simulink model "Test - Copy"  (R2019b)
settings: Solver=FixedStepAuto  StartTime=0.0  StopTime=10.0  FixedStep=0.005  RelTol=1e-3
undefined symbols (not defined in the file or in its folder): obj
settings Model: Creator=mecha  LastModifiedBy=mecha

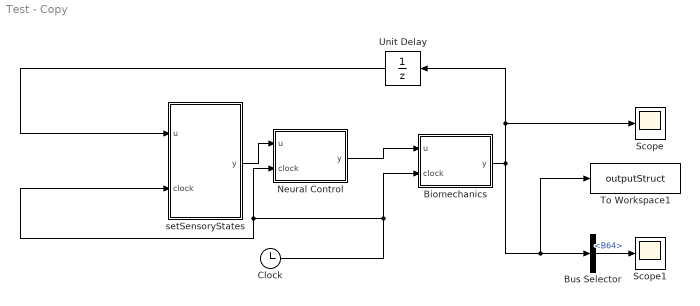
== system Test - Copy ==
  Biomechanics : MATLAB Function  TreatAsAtomicUnit=on
  Bus Selector : BusSelector  OutputSignals=B64
  Clock : Clock
  Neural Control : MATLAB Function  TreatAsAtomicUnit=on
  Scope : Scope
  Scope1 : Scope
  To Workspace1 : ToWorkspace  VariableName=outputStruct  SaveFormat=Timeseries  SampleTime=-1
  Unit Delay : UnitDelay  InitialCondition=obj  SampleTime=-1  HasFrameUpgradeWarning=on
  setSensoryStates : MATLAB Function  TreatAsAtomicUnit=on
  wires:
  Clock/1 -> Neural Control/2(clock), setSensoryStates/2(clock), Biomechanics/2(clock)
  Neural Control/1(y) -> Biomechanics/1(u)
  Biomechanics/1(y) -> Scope/1, Unit Delay/1, To Workspace1/1, Bus Selector/1
  setSensoryStates/1(y) -> Neural Control/1(u)
  Unit Delay/1 -> setSensoryStates/1(u)
  Bus Selector/1 -> Scope1/1  "<B64>"

== matlab function Test - Copy/Biomechanics ==
  data: u input Bus: AplysiaBus; y output Bus: AplysiaBus; clock input
function y = fcn(u, clock)
y=u;
%% Initialize internal tracking variables
tc=clock;
x_gh = u.x_g-u.x_h;
%initialize to avoid validation error upon build
F_f_g = 0;
F_f_h=0;
A11=0;
A12=0;
A21=0;
A22=0;
B1=0;
B2=0;
%% Biomechanics

%% Grasper Forces
%all forces in form F = Ax+b
F_I2 = u.max_I2*u.T_I2*[1,-1]*[u.x_h;u.x_g] + u.max_I2*u.T_I2*1; %FI2 = FI2_max*T_I2*(1-(xg-xh))
F_I3 = u.max_I3*u.T_I3*[-1,1]*[u.x_h;u.x_g]-u.max_I3*u.T_I3*0; %FI3 = FI3_max*T_I3*((xg-xh)-0)
F_hinge = (x_gh>0.5)*u.max_hinge*u.T_hinge*[-1,1]*[u.x_h;u.x_g]-(x_gh>0.5)*u.max_hinge*u.T_hinge*0.5; %F_hinge = [hinge stretched]*F_hinge_Max*T_hinge*((xg-xh)-0.5)
F_sp_g = u.K_sp_g*[1,-1]*[u.x_h;u.x_g]+u.K_sp_g*u.x_gh_ref; %F_sp,g = K_g((xghref-(xg-xh))

F_I4 = u.max_I4*u.P_I4;
F_I3_ant = u.max_I3ant*u.P_I3_anterior*[1,-1]*[u.x_h;u.x_g]+u.max_I3ant*u.P_I3_anterior*1;%: pinch force

%calculate F_f for grasper
if(u.fixation_type == 0) %object is not fixed to a contrained surface
    %F_g = F_I2+F_sp_g-F_I3-F_hinge; %if the object is unconstrained it does not apply a resistive force back on the grasper. Therefore the force is just due to the muscles

    A2 = 1/u.c_g*(u.max_I2*u.T_I2*[1,-1]+u.K_sp_g*[1,-1]-u.max_I3*u.T_I3*[-1,1]-u.max_hinge*u.T_hinge*(x_gh>0.5)*[-1,1]);
    B2 = 1/u.c_g*(u.max_I2*u.T_I2*1+u.K_sp_g*u.x_gh_ref+u.max_I3*u.T_I3*0+(x_gh>0.5)*u.max_hinge*u.T_hinge*0.5);

    A21 = A2(1);
    A22 = A2(2);

    %the force on the object is approximated based on the friction
    if(abs(F_I2+F_sp_g-F_I3-F_hinge) <= abs(u.mu_s_g*F_I4)) % static friction is true
        %disp('static')
        F_f_g = -u.sens_mechanical_grasper*(F_I2+F_sp_g-F_I3-F_hinge);
        y.grasper_friction_state = 1;
    else
        %disp('kinetic')
        F_f_g = u.sens_mechanical_grasper*u.mu_k_g*F_I4;
        %specify sign of friction force
        F_f_g = -(F_I2+F_sp_g-F_I3-F_hinge)/abs(F_I2+F_sp_g-F_I3-F_hinge)*F_f_g;
        y.grasper_friction_state = 0;
    end

elseif (u.fixation_type == 1) %object is fixed to a contrained surface
    if u.unbroken
        if(abs(F_I2+F_sp_g-F_I3-F_hinge) <= abs(u.mu_s_g*F_I4)) % static friction is true
            %disp('static')
            F_f_g = -u.sens_mechanical_grasper*(F_I2+F_sp_g-F_I3-F_hinge);
            %F_g = F_I2+F_sp_g-F_I3-F_hinge + F_f_g;
            y.grasper_friction_state = 1;

            %identify matrix components for semi-implicit integration
            A21 = 0;
            A22 = 0;
            B2 = 0;

        else
            %disp('kinetic')
            F_f_g = -sign(F_I2+F_sp_g-F_I3-F_hinge)*u.sens_mechanical_grasper*u.mu_k_g*F_I4;
            %specify sign of friction force
            %F_g = F_I2+F_sp_g-F_I3-F_hinge + F_f_g;
            y.grasper_friction_state = 0;


            %identify matrix components for semi-implicit integration
            A2 = 1/u.c_g*(u.max_I2*u.T_I2*[1,-1]+u.K_sp_g*[1,-1]-u.max_I3*u.T_I3*[-1,1]-u.max_hinge*u.T_hinge*(x_gh>0.5)*[-1,1]);
            B2 = 1/u.c_g*(u.max_I2*u.T_I2*1+u.K_sp_g*u.x_gh_ref+u.max_I3*u.T_I3*0+(x_gh>0.5)*u.max_hinge*u.T_hinge*0.5+F_f_g);

            A21 = A2(1);
            A22 = A2(2);

        end
    else
        %F_g = F_I2+F_sp_g-F_I3-F_hinge; %if the object is unconstrained it does not apply a resistive force back on the grasper. Therefore the force is just due to the muscles

        A2 = 1/u.c_g*(u.max_I2*u.T_I2*[1,-1]+u.K_sp_g*[1,-1]-u.max_I3*u.T_I3*[-1,1]-u.max_hinge*u.T_hinge*(x_gh>0.5)*[-1,1]);
        B2 = 1/u.c_g*(u.max_I2*u.T_I2*1+u.K_sp_g*u.x_gh_ref+u.max_I3*u.T_I3*0+(x_gh>0.5)*u.max_hinge*u.T_hinge*0.5);

        A21 = A2(1);
        A22 = A2(2);

        %the force on the object is approximated based on the friction
        if(abs(F_I2+F_sp_g-F_I3-F_hinge) <= abs(u.mu_s_g*F_I4)) % static friction is true
            %disp('static')
            F_f_g = -u.sens_mechanical_grasper*(F_I2+F_sp_g-F_I3-F_hinge);
            y.grasper_friction_state = 1;
        else
            %disp('kinetic')
            F_f_g = u.sens_mechanical_grasper*u.mu_k_g*F_I4;
            %specify sign of friction force
            F_f_g = -(F_I2+F_sp_g-F_I3-F_hinge)/abs(F_I2+F_sp_g-F_I3-F_hinge)*F_f_g;
            y.grasper_friction_state = 0;
        end
    end
end
%[j*dt position_grasper_relative I2 F_sp I3 hinge GrapserPressure_last F_g]

%% Body Forces
%all forces in the form F = Ax+b
F_sp_h = u.K_sp_h*[-1,0]*[u.x_h;u.x_g]+u.x_h_ref*u.K_sp_h;
%all muscle forces are equal and opposite
if(u.fixation_type == 0)     %object is not constrained
    %F_h = F_sp_h; %If the object is unconstrained it does not apply a force back on the head. Therefore the force is just due to the head spring.

    A1 = 1/u.c_h*u.K_sp_h*[-1,0];
    B1 = 1/u.c_h*u.x_h_ref*u.K_sp_h;

    A11 = A1(1);
    A12 = A1(2);

    if(abs(F_sp_h+F_f_g) <= abs(u.mu_s_h*F_I3_ant)) % static friction is true
        %disp('static2')
        F_f_h = -u.sens_mechanical_grasper*(F_sp_h+F_f_g); %only calculate the force if an object is actually present
        y.jaw_friction_state = 1;
    else
        %disp('kinetic2')
        F_f_h = -sign(F_sp_h+F_f_g)*u.sens_mechanical_grasper*u.mu_k_h*F_I3_ant; %only calculate the force if an object is actually present
        y.jaw_friction_state = 0;
    end
elseif (u.fixation_type == 1)
    %calcuate friction due to jaws
    if u.unbroken %if the seaweed is intact
        if(abs(F_sp_h+F_f_g) <= abs(u.mu_s_h*F_I3_ant)) % static friction is true
            %disp('static2')
            F_f_h = -u.sens_mechanical_grasper*(F_sp_h+F_f_g); %only calculate the force if an object is actually present
            %F_h = F_sp_h+F_f_g + F_f_h;
            y.jaw_friction_state = 1;

            A11 = 0;
            A12 = 0;
            B1 = 0;

        else
            %disp('kinetic2')
            F_f_h = -sign(F_sp_h+F_f_g)*u.sens_mechanical_grasper*u.mu_k_h*F_I3_ant; %only calculate the force if an object is actually present
            %F_h = F_sp_h+F_f_g + F_f_h;

            y.jaw_friction_state = 0;

            if (y.grasper_friction_state == 1) %object is fixed and grasper is static  
            % F_f_g = -mechanical_in_grasper*(F_I2+F_sp_g-F_I3-F_Hi);
                A1 = 1/u.c_h*(u.K_sp_h*[-1,0]+(-u.sens_mechanical_grasper*(u.max_I2*u.T_I2*[1,-1]+u.K_sp_g*[1,-1]-u.max_I3*u.T_I3*[-1,1]-u.max_hinge*u.T_hinge*(x_gh>0.5)*[-1,1]))...
                    -sign(F_sp_h+F_f_g)*u.sens_mechanical_grasper*u.mu_k_h*u.max_I3ant*u.P_I3_anterior*[1,-1]);
                B1 = 1/u.c_h*(u.x_h_ref*u.K_sp_h+(-u.sens_mechanical_grasper*(u.max_I2*u.T_I2*1+u.K_sp_g*u.x_gh_ref+u.max_I3*u.T_I3*0+(x_gh>0.5)*u.max_hinge*u.T_hinge*0.5))...
                    -sign(F_sp_h+F_f_g)*u.sens_mechanical_grasper*u.mu_k_h*u.max_I3ant*u.P_I3_anterior*1);

            else %both are kinetic
            %F_f_g = -sign(F_I2+F_sp_g-F_I3-F_Hi)*mechanical_in_grasper*mu_k_g*F_I4;
                A1 = 1/u.c_h*(u.K_sp_h*[-1,0]-sign(F_sp_h+F_f_g)*u.sens_mechanical_grasper*u.mu_k_h*u.max_I3ant*u.P_I3_anterior*[1,-1]);
                B1 = 1/u.c_h*(u.x_h_ref*u.K_sp_h-sign(F_I2+F_sp_g-F_I3-F_hinge)*u.sens_mechanical_grasper*u.mu_k_g*F_I4...
                    -sign(F_sp_h+F_f_g)*u.sens_mechanical_grasper*u.mu_k_h*u.max_I3ant*u.P_I3_anterior*1);                
            end
            A11= A1(1);
            A12 = A1(2);
        end
    else % if the seaweed is broken the jaws act as if unconstrained
        if(abs(F_sp_h+F_f_g) <= abs(u.mu_s_h*F_I3_ant)) % static friction is true
        %disp('static2')
            F_f_h = -u.sens_mechanical_grasper*(F_sp_h+F_f_g); %only calculate the force if an object is actually present
            y.jaw_friction_state = 1;
        else
            %disp('kinetic2')
            F_f_h = -sign(F_sp_h+F_f_g)*u.sens_mechanical_grasper*u.mu_k_h*F_I3_ant; %only calculate the force if an object is actually present
            y.jaw_friction_state = 0;
        end

        A1 = 1/u.c_h*u.K_sp_h*[-1,0];
        B1 = 1/u.c_h*u.x_h_ref*u.K_sp_h;

        A11 = A1(1);
        A12 = A1(2);
        y.jaw_friction_state = 0;

    end
end
%[position_buccal_last F_h F_sp I3 hinge force_pinch F_H]


%% Integrate body motions
%uncomment to remove periphery
%F_g = 0;
%F_H = 0;

A = [A11,A12;A21,A22];
B = [B1;B2];

x_last = [u.x_h;u.x_g];

x_new = 1/(1-u.TimeStep*trace(A))*((eye(2)+u.TimeStep*[-A22,A12;A21,-A11])*x_last+u.TimeStep*B);

y.x_g = x_new(2); 
y.x_h = x_new(1);

%% calculate force on object
y.force_on_object = F_f_g+F_f_h;

%check if seaweed is broken
if (u.fixation_type ==1)
    if (y.force_on_object>u.seaweed_strength)
        u.unbroken = 0;
    end
    %check to see if a new cycle has started
    x_gh_next = y.x_g-y.x_h;

    if (~u.unbroken && x_gh <0.3 && x_gh_next>x_gh)%x_gh<0.3)
       y.unbroken = 1; 
    end
y.force_on_object= y.unbroken*y.force_on_object;
end










end

== matlab function Test - Copy/Neural Control ==
  data: u input Bus: AplysiaBus; y output Bus: AplysiaBus; clock input
function y = fcn(u, clock)
y=u
%% Initialize internal tracking variables
tc=clock;

%j=1;

% u.CBI3_stimON = 0;
% u.CBI3_stimOFF = 0;
% u.CBI3_refractory = 0;
% u.B40B30_offTime = 0;
% u.unbroken = 1; %tracking variable to keep track of seaweed being broken off during feeding



x_gh = u.x_g-u.x_h;

%% Update Metacerebral cell: 
% assume here feeding arousal continues
% indefinitely, once started. 
%{
MCC is active IF
    General Food arousal is on
%}

y.MCC=u.MCC;

%% Update CBI-2
%{
CBI2 is active IF
    MCC is on 
    AND (
        (Mechanical Stimulation at Lips AND Chemical Stimulation at Lips AND No mechanical stimuli in grasper)
        OR 
        (Mechanical in grasper and no Chemical Stimulation at Lips)
        OR
        (B4/B5 is firing strongly (>=2)))
%}

%CBI2 - updated 6/7/2020
%with hypothesized connections from B4/B5
if (u.use_hypothesized_connections ==1)
     y.CBI2 = (u.stim_CBI2==0)*... if electrode above CBI-2 is off, do this:
         u.MCC*(~u.B64)*((u.sens_mechanical_lips && u.sens_chemical_lips &&(~u.sens_mechanical_grasper))||(u.sens_mechanical_grasper &&(~u.sens_chemical_lips))||(u.B4B5>=2))+...
         (u.stim_CBI2==1);
else
%without hypothesized connections from B4/B5
    y.CBI2 = (u.stim_CBI2==0)*... if electrode above CBI-2 is off, do this:
        u.MCC*(~u.B64)*((u.sens_mechanical_lips && u.sens_chemical_lips &&(~u.sens_mechanical_grasper))||(u.sens_mechanical_grasper&&(~u.sens_chemical_lips)))+...
        (u.stim_CBI2==1);
end

%% Update CBI-3
% requires stimuli_mech_last AND stimuli_chem_last
%{
CBI3 is active IF
    MCC is on
    AND
    Mechanical Simulation at Lips
    AND
    Chemical Stimulation at Lips
    AND
    B4/B5 is NOT firing strongly
    AND
    CBI3 is NOT in a refractory period
%}

%CBI3 can experieince a refractory period following strong inhibition from B4/B5
%check if a refractory period is occuring

%modified to only turn on refreactory after the strong stimulation
if((u.B4B5>=2) && (y.CBI3_stimON==0))
   y.CBI3_stimON = tc;   
   %CBI3_refractory = 1;
end
if ((y.CBI3_stimON ~=0) && (u.B4B5<2))
   y.CBI3_refractory = 1;
   y.CBI3_stimOFF = tc;  
   y.CBI3_stimON = 0;    
end 

if(y.CBI3_refractory && clock<(y.CBI3_stimOFF+u.refractory_CBI3/1000)) %modified [RS]
   y.CBI3_refractory = 1; 
else
    y.CBI3_stimOFF = 0;
    y.CBI3_refractory = 0; 
end


%CBI3 - updated 6/7/2020    
%with hypothesized connections from B4/B5    
if (u.use_hypothesized_connections ==1)
    y.CBI3 = u.MCC*(u.sens_mechanical_lips*u.sens_chemical_lips)*((u.B4B5<2))*(~y.CBI3_refractory);   
else
%without hypothesized connections from B4/B5  
    y.CBI3 = u.MCC*(u.sens_mechanical_lips*u.sens_chemical_lips); 
end



%% Update CBI4 - added 2/27/2020
%{
CBI4 is active IF Â– mediates swallowing and rejection
    MCC is on
    AND
        (Mechanical Stimulation at Lips
        OR
        Chemical Stimulation at Lips)
    AND
    Mechanical Stimulation in grasper
%}
y.CBI4 = u.MCC*(u.sens_mechanical_lips || u.sens_chemical_lips)*u.sens_mechanical_grasper;

%% Update B64
% list of inputs
% Protraction threshold excites
% grasper pressure excites - still figuring out how to implement
% retraction threshold inhibits
% B31/32 inhibits

%If there is mechanical and chemical stimuli at the lips and there is
%seaweed in the grasper -> swallow

%If there is mechanical and chemical stimuli at the lips and there is
%NOT seaweed in the grasper -> bite

%If there is not chemical stimuli at the lips but there is mechanical
%stimuli ->reject

%{
B64 is active IF
    MCC is on
    AND
    IF CBI3 is active (ingestion)
        IF mechanical stimulation is in grasper (swallowing)
            Relative Grasper Position is Greater than B64 Swallowing Protraction threshold
        IF mechanical stimulation is NOT in grasper (biting)
            Relative Grasper Position is Greater than B64 Biting Protraction threshold
    IF CBI3 is NOT active (rejection)
        Relative Grasper Position is Greater than B64 Rejection Protraction threshold
    AND
    B31/B32 is NOT active
    AND
    IF CBI3 is active (ingestion)
        IF mechanical stimulation is in grasper (swallowing)
            NOT (Relative Grasper Position is less than B64 Swallow Retraction threshold)
        IF mechanical stimulation is NOT in grasper (biting)
            NOT(Relative Grasper Position is less than B64 Biting Retraction threshold)
    IF CBI3 is NOT active (rejection)
        NOT(Relative Grasper Position is less than B64 Rejection Retraction threshold)
%}

B64_proprioception = (u.CBI3*(... % checks protraction threshold - original 0.5
                                (  u.sens_mechanical_grasper *(x_gh>u.thresh_B64_swallow_protract))||...
                                ((~u.sens_mechanical_grasper)*(x_gh>u.thresh_B64_bite_protract))))...
                            ||...
                                ((~u.CBI3)                   *(x_gh>u.thresh_B64_reject_protract));

%B64
y.B64=u.MCC*(~u.B31B32)*... % update B64
    B64_proprioception;

%% Update B4/B5: 
%{
B4/B5 is active IF
    MCC is ON
    AND
    IF stimulating electrode is off
        Strongly firing IF CBI3 is NOT active (rejection)
            AND
            B64 is active (retraction)
            AND
            Relative grasper position is greater than B4/B5 threshold (early retraction)
        weakly firing IF CBI3 is active (ingestion)
            AND
            B64 is active (retraction)
            AND
            mechanical stimulation is in grasper (swallowing)
    If stimulating electrode is on
        Activity is set to 2 to designate strong firing
%}

%B4B5
y.B4B5=u.MCC*...
            ((~u.stim_B4B5)*... % when B4/B5 electrode is off
                (2*(~u.CBI3)*...% if egestion
                    u.B64*(x_gh>u.thresh_B4B5_protract)) +... 
                ((u.CBI3)*(u.sens_mechanical_grasper)*u.B64))... % if swallowing
    +2*u.stim_B4B5; % when B4/B5 electrode is on (and +1) then turn B4/B5 on to "emergency" mode

%% Update B20 - updated 2/27/2020
% Not active if CB1-3 is on (strongly inhibited)
%excited by CBI2 but excitation is weaker than inhibition from CBI3
%{
(CBI2 is active
    OR	
    CBI4 is active
    OR
    B63 (B31/32) is active)
        AND
        CBI3 is NOT active
        AND
        B64 is NOT active

%}
y.B20 = u.MCC*((u.CBI2 || u.CBI4) || u.B31B32)*(~u.CBI3)*(~u.B64);

%% Update B40/B30
%{
B40/B30 is active IF
    MCC is ON
    AND
    (CBI2 is active
    OR 
    CBI4 is active
    OR 
    B63 (B31/32) is active)
    AND 
    B64 is not active
%}

% B30/B40 have a fast inhibitory and slow excitatory connection with
% B8a/b. To accomodate this, we track when B30/B40 goes from a active
% state to a quiescent state 

y.B40B30 = u.MCC*((u.CBI2 || u.CBI4) || u.B31B32)*(~u.B64);

%check if B30/B40 has gone from active to quiescent
if((u.B40B30 ==1) && (y.B40B30==0))
   y.B40B30_offTime = tc;
end

%% Update B31/B32: -updated 2/27/2020
% activated if grasper retracted enough, inhibited if
% pressure exceeds a threshold or grasper is protracted far enough
%{
B31/B32 is active IF
    MCC is ON
    AND
    IF CBI3 is active (ingestion)
        B64 is NOT active (protraction)
        AND
            Graper pressure is less than half of its maximum (open)
            OR
            CBI2 is active (biting)
        AND
        IF B31/B32 is NOT firing (switching to protraction)
            The relative grasper position is less than the retraction threshold
        IF B31/B32 is firing (protraction)
            The relative grasper position is less than the protraction threshold
    IF CBI3 is NOT active (rejection)
        B64 is NOT active (protraction)
        AND
        Grasper Pressure is greater than a quarter of the maximum (closing or closed)
        AND
            CBI2 is active
            OR
            CBI4 is active
        AND
        IF B31/B32 is NOT firing (switching to protraction)
            The relative grasper position is less than the retraction threshold
        IF B31/B32 is firing (protraction)
            The relative grasper position is less than the protraction threshold
%}

%B31/B32s thresholds may vary for different behaviors. These are set
%here
if (u.sens_mechanical_grasper && u.CBI3) %swallowing
    on_thresh = u.thresh_B31_swallow_on;
    off_thresh = u.thresh_B31_swallow_off;
elseif (u.sens_mechanical_grasper && (~u.CBI3)) %rejection
    on_thresh = u.thresh_B31_reject_on;
    off_thresh = u.thresh_B31_reject_off;
else %biting
    on_thresh = u.thresh_B31_bite_on;
    off_thresh = u.thresh_B31_bite_off;        
end

y.B31B32=u.MCC*(...
    u.CBI3*... %if ingestion
        ((~u.B64)*((u.P_I4<(1/2))||u.CBI2)*... 
            ((~u.B31B32)*(x_gh<off_thresh)+...
               u.B31B32 *(x_gh<on_thresh)))+...
  (~u.CBI3)*... %if egestion
        ((~u.B64)*(u.P_I4>(1/4))*(u.CBI2||u.CBI4)*...
            ((~u.B31B32)*(x_gh<off_thresh)+...
               u.B31B32 *(x_gh<on_thresh))));

%% Update B6/B9/B3: 
% activate once pressure is high enough in ingestion, or low enough in
% rejection
%{
NEW VERSION:
B6/B9/B3 is active IF
    MCC is active
    AND
    B4/B5 is NOT firing strongly
    AND
    IF CBI3 is active (ingestion)
        B64 is active (retraction)
        AND
        Grasper pressure is greater than B6/B3/B9 pressure threshold (closed)
    IF CBI3 is not active (rejection)
        B64 is active (retraction)
        AND
        Grasper pressure is less than B6/B3/B9 pressure threshold (open)
%}
%{
B6/B9/B3 is active IF
    MCC is active
    AND
    B64 is active (retraction)
    AND
    B4/B5 is NOT firing strongly
    AND (
    (CBI3 is active (ingestion)
     AND
     There is NOT mechanical stimulation in mouth (biting)
     AND
     Grasper pressure is greater than B6/B3/B9 biting pressure
     threshold (closed))
    OR
    (CBI3 is active (ingestion)
     AND
     There is mechanical stimulation in mouth (swallowing)
     AND
     Grasper pressure is greater than B6/B3/B9 swallowing pressure
     threshold (closed))
    OR
    (CBI3 is NOT active (rejection)
     AND
     Grasper pressure is NOT greater than B6/B3/B9 rejection pressure
     threshold (open))
    )
%}

%B6/B9/B3
y.B6B9B3= u.MCC*u.B64*(~(u.B4B5>=2))*(...
                (u.CBI3 && ~u.sens_mechanical_grasper)*... biting
                    (u.P_I4>u.thresh_B6B9B3_bite_pressure)...
                +...
                (u.CBI3 && u.sens_mechanical_grasper)*... swallowing
                    (u.P_I4>u.thresh_B6B9B3_swallow_pressure)...
                +...
                (~u.CBI3)*... rejection
                    (~(u.P_I4>u.thresh_B6B9B3_reject_pressure)));


%% Update B8a/b
% active if excitation from B6/B9/B3 plus protracted
% sensory feedback exceeds threshold of 1.9, and not inhibited by
% either B31/B32 or by sensory feedback from being retracted. If B4/B5 is
% highly excited (activation level is 2 instead of just 1) then shut
% down B8a/b.
%{
B8a/b is active IF
    MCC is on
    AND
        B64 is active
        OR
        B40/B30 is NOT active
        OR
        B20 is active
    AND
    B4/B5 is not active
    AND
        B20 is active
        OR
        B31/B32 is NOT active
%}

%B8a/b recieves slow exitatory input from B30/B40 functionally this
%causes strong firing immediatly following B30/B40 cessation in biting
%and swallowing
if(u.B40B30==0 && clock<(y.B40B30_offTime+u.postActivityExcitation_B40B30/1000))
    B40B30_excite = 1; 
else
    B40B30_excite = 0; 
end

%B8a/b - updated 5/25/2020   
y.B8 = u.MCC*(~(u.B4B5>=2))*(...%B4/5 inhibits when strongly active
            u.CBI3*(... % if ingestion
                u.B20 || (B40B30_excite)*(~u.B31B32))+...
            (~u.CBI3)*(... % if rejection
                u.B20)); 

%% Update B7 - ONLY ACTIVE DURING EGESTION and BITING
% turn on as you get to peak protraction
%in biting this has a threshold that it stops applying effective force -
%biomechanics
%{
B7 is active IF
    ((CBI3 is NOT active (rejection)
    OR
    There is mechanical stimulation in mouth
    AND
        (The relative position of the grasper is greater than the rejection protraction threshold
        OR
        Grasper pressure is very high) (closed))
    OR
    (CBI3 is active
    AND
    There is NOT mechanical stimulation in mouth (biting)
    AND
        (The relative position of the grasper is greater than the bite protraction threshold
        OR
        Grasper pressure is very high) (closed))
%}
y.B7 = u.MCC*( ...
                  (((~u.CBI3) ||  (u.sens_mechanical_grasper))*((x_gh>=u.thresh_B7_reject_protract)||(u.P_I4>(.97)))) + ...
                  (  (u.CBI3  && (~u.sens_mechanical_grasper))*((x_gh>=u.thresh_B7_bite_protract)  ||(u.P_I4>(.97)))) ...
                  );

%% Update B38: 
% If already active, remain active until protracted past
% 0.5.  If inactive, become active if retracted to 0.1 or further. 
%{
B38 is active IF
    MCC is ON
    AND
    mechanical stimulation in the grasper (swallowing or rejection)
    AND
    IF CBI3 is active (ingestion)
        Relative grasper position is less than B38 ingestion threshold
    IF CBI3 is not active (rejection)
        Turn off B38
%}

%B38

y.B38=u.MCC*(u.sens_mechanical_grasper)*(...
    (u.CBI3)*(... % if CBI3 active do the following:
        ((x_gh)<u.thresh_B38_retract)));

%% Update I4: If food present, and grasper closed, then approaches
% max pressure 
y.P_I4=((u.tau_I4*u.P_I4+u.A_I4*u.TimeStep)/(u.tau_I4+u.TimeStep));%old -- keep this version
y.A_I4=((u.tau_I4*u.A_I4+u.B8*u.TimeStep)/(u.tau_I4+u.TimeStep));

%% Update pinch force: If food present, and grasper closed, then approaches
% max pressure
y.P_I3_anterior=(u.tau_I3anterior*u.P_I3_anterior+u.A_I3_anterior*u.TimeStep)/(u.tau_I3anterior+u.TimeStep);
y.A_I3_anterior=(u.tau_I3anterior*u.A_I3_anterior+(u.B38+u.B6B9B3)*u.TimeStep)/(u.tau_I3anterior+u.TimeStep);

%% Update I3 (retractor) activation: 
y.T_I3=(u.tau_I3*u.T_I3+u.TimeStep*u.A_I3)/(u.tau_I3+u.TimeStep);
y.A_I3=(u.tau_I3*u.A_I3+u.TimeStep*u.B6B9B3)/(u.tau_I3+u.TimeStep);

%% Update I2 (protractor) activation: 
y.T_I2=((u.tau_I2_ingestion*u.CBI3+u.tau_I2_egestion*(1-u.CBI3))*u.T_I2+u.TimeStep*u.A_I2)/((u.tau_I2_ingestion*u.CBI3+u.tau_I2_egestion*(1-u.CBI3))+u.TimeStep);
y.A_I2=((u.tau_I2_ingestion*u.CBI3+u.tau_I2_egestion*(1-u.CBI3))*u.A_I2+u.TimeStep*u.B31B32)/((u.tau_I2_ingestion*u.CBI3+u.tau_I2_egestion*(1-u.CBI3))+u.TimeStep);

%% Update Hinge activation: 
y.T_hinge=(u.tau_hinge*u.T_hinge+u.TimeStep*u.A_hinge)/(u.tau_hinge+u.TimeStep);%new
y.A_hinge=(u.tau_hinge*u.A_hinge+u.TimeStep*u.B7)/(u.tau_hinge+u.TimeStep);




%y=u;
end

== matlab function Test - Copy/setSensoryStates ==
  data: u input Bus: AplysiaBus; y output Bus: AplysiaBus; clock input
function y = fcn(u, clock)
y=u
%% Initialize internal tracking variables
tc=clock;
% switchBehavior = sens(1);
% behavior_1 = sens(2);
% behavior_2 = sens(3);
% t_switch = sens(4);

if (u.switchBehavior == 0)
    
    if (u.behavior_1==1) %bite
        y.sens_chemical_lips = 1;
        y.sens_mechanical_lips = 1;
        y.sens_mechanical_grasper = 0;
        y.fixation_type = 0;
    elseif (u.behavior_1==2) %swallow
        y.sens_chemical_lips = 1;
        y.sens_mechanical_lips = 1;
        y.sens_mechanical_grasper = 1;
        y.fixation_type = 1;
    elseif (u.behavior_1==2) %reject
        y.sens_chemical_lips = 0;
        y.sens_mechanical_lips = 1;
        y.sens_mechanical_grasper = 1;
        y.fixation_type = 0;
    end

elseif (u.switchBehavior == 1)
    



    if (u.behavior_1==1) %bite
        y.sens_chemical_lips = 1;
        y.sens_mechanical_lips = 1;
        y.sens_mechanical_grasper = 0;
        y.fixation_type = 0;
    elseif (u.behavior_1==2) %swallow
        y.sens_chemical_lips = 1;
        y.sens_mechanical_lips = 1;
        y.sens_mechanical_grasper = 1;
        y.fixation_type = 1;
    elseif (u.behavior_1==2) %reject
        y.sens_chemical_lips = 0;
        y.sens_mechanical_lips = 1;
        y.sens_mechanical_grasper = 1;
        y.fixation_type = 0;
    end

    if (tc> u.t_switch)
        
        if (u.behavior_1==1) %bite
            y.sens_chemical_lips = 1; %1
            y.sens_mechanical_lips = 1; %1
            y.sens_mechanical_grasper = 0; %0
            y.fixation_type = 0; %0

        elseif (u.behavior_1==2) %swallow
            y.sens_chemical_lips = 1;
            y.sens_mechanical_lips = 1;
            y.sens_mechanical_grasper = 1;
            y.fixation_type = 1;
            
       
        elseif (u.behavior_1==2) %reject
            y.sens_chemical_lips = 0;
            y.sens_mechanical_lips = 1;
            y.sens_mechanical_grasper = 1;
            y.fixation_type = 0;
  
        end
    end
end



%y=u;
end
